simulink model "model3"  (R2024a)
settings: Solver=VariableStepAuto  StartTime=0.0  StopTime=10.0  RelTol=1e-3
values from neighbouring files (symbols this model uses):
  A = 1    [modelSave.m]    (also in script3.m = [ 5  -9  -7   1)
  B = [3; 3; 1; 3]    [script3.m]
  C = 1    [modelSave.m]    (also in script3.m = [ 2  -2   2   2)
  D = 1    [modelSave.m]    (also in script3.m = [4; 1])
  K = 1    [modelSave.m]    (also in script3.m = -a_bar * inv(Aa) * inv(Uc))
  L = 1    [modelSave.m]    (also in script3.m = V * L_tilde)
settings Model: Creator=eva  LastModifiedBy=eva

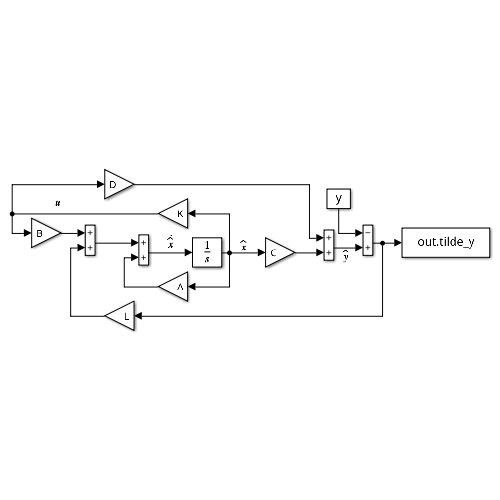
[thumbnail: Simulink's stored preview of the top-level diagram]
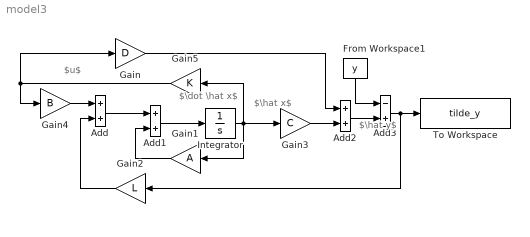
== system model3 ==
  note: $\hat x$
  note: $\dot \hat x$
  note: $u$
  note: $\hat y$
  Add : Sum
  Add1 : Sum
  Add2 : Sum
  Add3 : Sum  Inputs=-+
  From Workspace1 : FromWorkspace  VariableName=y
  Gain : Gain  Gain=D
  Gain1 : Gain  Gain=A
  Gain2 : Gain  Gain=L
  Gain3 : Gain  Gain=C
  Gain4 : Gain  Gain=B
  Gain5 : Gain  Gain=K
  Integrator : Integrator
  To Workspace : ToWorkspace  VariableName=tilde_y  SaveFormat=Timeseries  SampleTime=-1
  wires:
  Integrator/1 -> Gain3/1, Gain5/1, Gain1/1
  Gain1/1 -> Add1/2
  Add/1 -> Add1/1
  Add1/1 -> Integrator/1
  Gain3/1 -> Add2/2
  Gain/1 -> Add2/1
  Gain4/1 -> Add/1
  Gain5/1 -> Gain/1, Gain4/1
  Add2/1 -> Add3/2
  From Workspace1/1 -> Add3/1
  Add3/1 -> To Workspace/1, Gain2/1
  Gain2/1 -> Add/2
